simulink model "db"  (R2023b)
settings: Solver=VariableStepAuto  StartTime=0.0  StopTime=tu  RelTol=1e-3
values from neighbouring files (symbols this model uses):
  A = 5    [Tarea_2.m]
  deltad = Xvs0 - 0.1    (= 0.4)    [Tarea_2.m]
  deltau = u0 - 10    [Tarea_2.m]
  g = 9.81    [Tarea_2.m]
  H0 = 2.5    [Tarea_2.m]
  K1 = (2 / (Xvs0 * Kvs)) * sqrt(H0 /(rho * g))    [Tarea_2.m]
  K2 = -2 * H0/Xvs0    (= -10)    [Tarea_2.m]
  Kt = 100/3.25    (= 30.7692307692)    [Tarea_2.m]
  Kvc = Qemax/100    [Tarea_2.m]
  Kvs = 0.001    [Tarea_2.m]
  rho = 1027    [Tarea_2.m]
  steptimed = 1500    [Tarea_2.m]
  steptimeu = 100    [Tarea_2.m]
  T = (2 * A / (Xvs0 * Kvs)) * sqrt(H0 /(rho * g))    [Tarea_2.m]
  u0 = Qe0/Kvc    [Tarea_2.m]
  Xvs0 = 0.5    [Tarea_2.m]
settings Model: Creator=roger  LastModifiedBy=roger

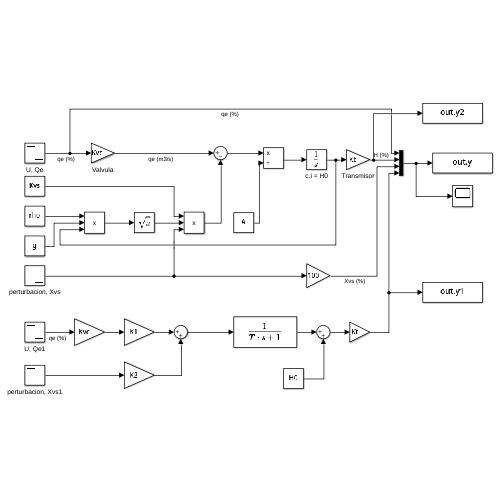
[thumbnail: Simulink's stored preview of the top-level diagram]
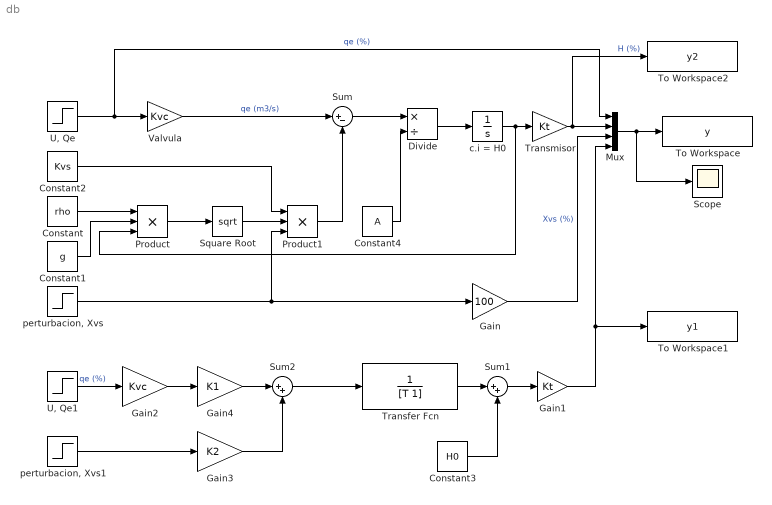
== system db ==
  Constant : Constant  Value=rho
  Constant1 : Constant  Value=g
  Constant2 : Constant  Value=Kvs
  Constant3 : Constant  Value=H0
  Constant4 : Constant  Value=A
  Divide : Product  Inputs=*/
  Gain : Gain  Gain=100
  Gain1 : Gain  Gain=Kt
  Gain2 : Gain  Gain=Kvc
  Gain3 : Gain  Gain=K2
  Gain4 : Gain  Gain=K1
  Mux : Mux
  Product : Product  Inputs=3
  Product1 : Product  Inputs=3
  Scope : Scope
  Square Root : Sqrt
  Sum : Sum  Inputs=|+-
  Sum1 : Sum  Inputs=|++
  Sum2 : Sum  Inputs=|++
  To Workspace : ToWorkspace  VariableName=y  SaveFormat=Timeseries  SampleTime=-1
  To Workspace1 : ToWorkspace  VariableName=y1  SaveFormat=Timeseries  SampleTime=-1
  To Workspace2 : ToWorkspace  VariableName=y2  SaveFormat=Timeseries  SampleTime=-1
  Transfer Fcn : TransferFcn  Denominator=[T 1]
  Transmisor : Gain  Gain=Kt
  "U, Qe" : Step  Time=steptimeu  Before=u0  After=deltau  SampleTime=0
  "U, Qe1" : Step  Time=steptimeu  Before=u0  After=deltau  SampleTime=0
  Valvula : Gain  Gain=Kvc
  c.i = H0 : Integrator  InitialCondition=H0
  "perturbacion, Xvs" : Step  Time=steptimed  Before=Xvs0  After=deltad  SampleTime=0
  "perturbacion, Xvs1" : Step  Time=steptimed  Before=Xvs0  After=deltad  SampleTime=0
  wires:
  Constant/1 -> Product/1
  Product/1 -> Square Root/1
  Constant2/1 -> Product1/1
  Square Root/1 -> Product1/2
  "U, Qe"/1 -> Mux/1, Valvula/1  "qe (%)"
  Valvula/1 -> Sum/1  "qe (m3/s)"
  Divide/1 -> c.i = H0/1
  Product1/1 -> Sum/2
  "perturbacion, Xvs"/1 -> Product1/3, Gain/1
  c.i = H0/1 -> Product/3, Transmisor/1
  Mux/1 -> To Workspace/1, Scope/1
  Transmisor/1 -> To Workspace2/1, Mux/2  "H (%)"
  Gain/1 -> Mux/3  "Xvs (%)"
  Sum/1 -> Divide/1
  Constant4/1 -> Divide/2
  Constant1/1 -> Product/2
  Gain2/1 -> Gain4/1
  Gain4/1 -> Sum2/1
  Sum2/1 -> Transfer Fcn/1
  Gain3/1 -> Sum2/2
  Transfer Fcn/1 -> Sum1/1
  Constant3/1 -> Sum1/2
  Sum1/1 -> Gain1/1
  Gain1/1 -> To Workspace1/1, Mux/4
  "U, Qe1"/1 -> Gain2/1  "qe (%)"
  "perturbacion, Xvs1"/1 -> Gain3/1
